simulink model "threshingDrum"  (R2025b)
settings: Solver=FixedStepDiscrete  StartTime=0.0  StopTime=10.0  FixedStep=0.1  RelTol=1e-3
values from neighbouring files (symbols this model uses):
  nDrum = 1000    [Script.m]
settings Model: Creator=Atread  LastModifiedBy=andr
settings OptimizationCC: DefaultParameterBehavior=Inlined  UseDivisionForNetSlopeComputation=on  GainParamInheritBuiltInType=on  UseFloatMulNetSlope=on  InlineInvariantSignals=on  PassReuseOutputArgsAs=Individual arguments  ZeroExternalMemoryAtStartup=off  ZeroInternalMemoryAtStartup=off  NoFixptDivByZeroProtection=on  EfficientFloat2IntCast=on  LifeSpan=1  OptimizeBlockOrder=speed  DifferentSizesBufferReuse=on  EfficientTunableParamExpr=on
settings DebuggingCC: ParameterTunabilityLossMsg=error  SFUnexpectedBacktrackingDiag=warning  SFNoUnconditionalDefaultTransitionDiag=warning
settings HardwareCC: ProdLongLongMode=on
settings SFSimCC: MATLABDynamicMemAlloc=off  SimTargetLang=C++  SimDLTargetLibrary=mkl-dnn
settings RTWCC: SystemTargetFile=ert.tlc  TemplateMakefile=ert_default_tmf  GenerateReport=on  BuildConfiguration=Debug  LaunchReport=on  TargetLang=C++  Description=Embedded Coder
settings CodeAppCC: ForceParamTrailComments=on  IgnoreCustomStorageClasses=off  OperatorAnnotations=on  SimulinkDataObjDesc=on  SFDataObjDesc=on  InsertBlockDesc=on  EnableCustomComments=on
settings ERTTargetCC: RootIOFormat=Structure reference  ERTCustomFileTemplate=example_file_process.tlc  ERTFilePackagingFormat=CompactWithDataFile  TargetLangStandard=C++20 (ISO)  GenerateSampleERTMain=on  IncludeMdlTerminateFcn=off  CombineSignalStateStructs=on  SuppressErrorStatus=on  SupportAbsoluteTime=off  CodeInterfacePackaging=C++ class  SubcomponentCodeInterfacePackaging=C++ class  SupportComplex=off

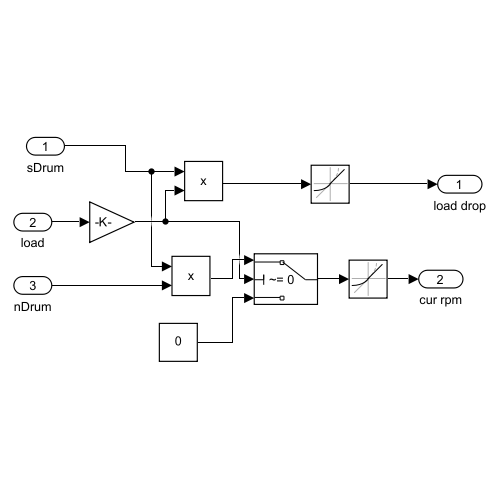
[thumbnail: Simulink's stored preview of the top-level diagram]
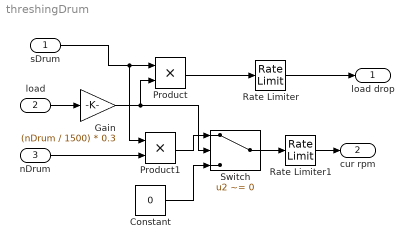
== system threshingDrum ==
  sDrum : Inport  OutDataTypeStr=boolean
  load : Inport  Port=2  OutDataTypeStr=double
  nDrum : Inport  Port=3  OutDataTypeStr=double
  Constant : Constant  Value=0
  Gain : Gain  Gain=(nDrum / 1500) * 0.3
  Product : Product  OutDataTypeStr=double
  Product1 : Product  OutDataTypeStr=double
  Rate Limiter : RateLimiter  RisingSlewLimit=250  FallingSlewLimit=-250  SampleTimeMode=inherited
  Rate Limiter1 : RateLimiter  RisingSlewLimit=350  FallingSlewLimit=-350  SampleTimeMode=inherited
  Switch : Switch  Criteria=u2 ~= 0  SaturateOnIntegerOverflow=off  InputSameDT=off
  load drop : Outport  OutDataTypeStr=double
  cur rpm : Outport  Port=2  OutDataTypeStr=double
  wires:
  Rate Limiter/1 -> load drop/1
  Product/1 -> Rate Limiter/1
  sDrum/1 -> Product/1, Product1/1
  load/1 -> Gain/1
  Gain/1 -> Switch/2, Product/2
  Rate Limiter1/1 -> cur rpm/1
  nDrum/1 -> Product1/2
  Switch/1 -> Rate Limiter1/1
  Product1/1 -> Switch/1
  Constant/1 -> Switch/3
